simulink model "INVERTER_Arduino"  (R2022b)
settings: Solver=FixedStepAuto  StartTime=0.0  StopTime=100e-3  FixedStep=samplerate  RelTol=1e-3  EnableMultiTasking=on
InitFcn:
  | addpath('Library_Subsystems')
  | 
  | samplerate = 10e-3;
  | samplerate_serial = 100e-3;
  | samplerate_udp = 100e-3;
  | 
  | fsw = 10000;
  | 
  | 
  | PWMclock = 100e6;
  | period = PWMclock/fsw/2;
libraries: arduinolib x3, simulink x2
settings Model: SimulationMode=external  ExtModeTrigDuration=2  Creator=ReiterTo  LastModifiedBy=ReiterTo
settings SolverCC: AlgebraicLoopSolver=TrustRegion  PositivePriorityOrder=on  AutoInsertRateTranBlk=on
settings DataIOCC: LimitDataPoints=on  MaxDataPoints=10000  InspectSignalLogs=on
settings OptimizationCC: DefaultParameterBehavior=Inlined  GainParamInheritBuiltInType=on  UseFloatMulNetSlope=on  InlineInvariantSignals=on  EnhancedBackFolding=on  StrengthReduction=on  PassReuseOutputArgsAs=Individual arguments  ZeroExternalMemoryAtStartup=off  ZeroInternalMemoryAtStartup=off  NoFixptDivByZeroProtection=on  EfficientFloat2IntCast=on  LifeSpan=1  MaxStackSize=64  BufferReusableBoundary=off  OptimizeBlockOrder=speed  OptimizationPriority=Speed  MultiThreadedLoops=on  EfficientTunableParamExpr=on
settings DebuggingCC: ParameterOverflowMsg=none  ParameterUnderflowMsg=error  ParameterPrecisionLossMsg=none  ParameterTunabilityLossMsg=error
settings HardwareCC: ProdBitPerPointer=32  ProdBitPerSizeT=32  ProdBitPerPtrDiffT=32  ProdLargestAtomicInteger=Long  ProdLargestAtomicFloat=Double  ProdWordSize=32  ProdHWDeviceType=ARM Compatible->ARM Cortex  UseEmbeddedCoderFeatures=off
settings SFSimCC: MATLABDynamicMemAlloc=off
settings RTWCC: Description=Embedded Coder  SystemTargetFile=ert.tlc  HardwareBoard=Arduino Nano 33 IoT  TLCOptions=-aInlineSetEventsForThisBaseRateFcn=TLC_FALSE -aSuppressMultiTaskScheduler=TLC_FALSE -aRateBasedStepFcn=1  TemplateMakefile=ert_default_tmf  Toolchain=Arduino ARM  BuildConfiguration=Faster Runs  CodeProfilingSaveOptions=MetricsOnly
settings CodeAppCC: ForceParamTrailComments=on  IgnoreCustomStorageClasses=off  OperatorAnnotations=on  SimulinkDataObjDesc=on  SFDataObjDesc=on  InsertBlockDesc=on
settings ERTTargetCC: TargetLangStandard=C99 (ISO)  SupportNonFinite=off  SupportNonInlinedSFcns=on  SupportVariableSizeSignals=on  ExtModeTransport=3  ExtModeStaticAlloc=on  ExtModeStaticAllocSize=8192  ExtModeMexFile=ext_xcp  ExtModeIntrfLevel=Level2 - Open

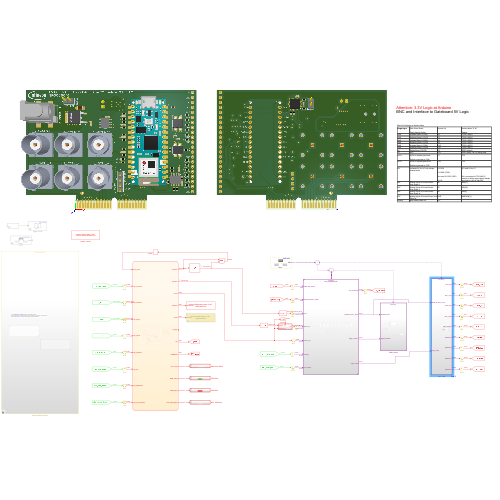
[thumbnail: Simulink's stored preview of the top-level diagram]
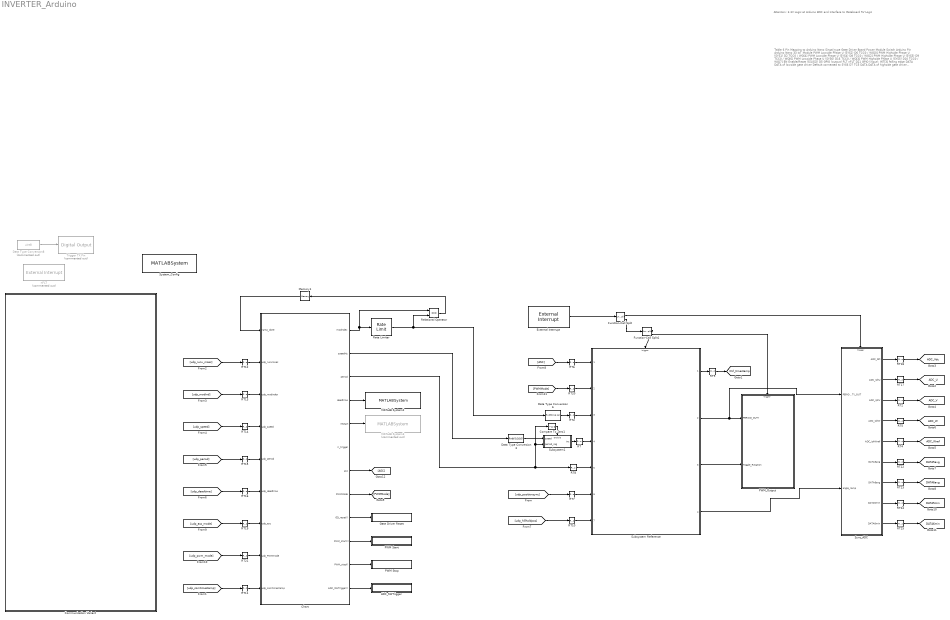
== system INVERTER_Arduino ==
  note: Attention: 3.3V Logic at Arduino
      | BNC and Interface to Gateboard 5V Logic
  note: Table 6 Pin Mapping to Arduino Nano
      | Singal type
      | Gate Driver Board
      | Power Module Switch
      | Arduino Pin
      |
      | Arduino Nano 33 IoT
      | Module
      |
      | PWM
      | Lowside Phase U (SYS2)
      | D6
      | TCC0 / WO[0]
      |
      | PWM
      | Highside Phase U (SYS1)
      | D2
      | TCC0 / WO[4]
      |
      | PWM
      | Lowside Phase U (SYS4)
      | D8
      | TCC0 / WO[2]
      |
      | PWM
      | Highside Phase U (SYS3)
      | D9
      | TCC0 / WO[6]
      |
      | PWM
      | Lowside Phase U (SYS6)
      | D16
      | TCC0 / WO[3]
      |
      | PWM
      | Highside Phase U (SYS5)
      | D10
      | TCC0 / WO[7]
      |
      | EN
      | Enable/Reset (SI1|SI2)
      | D5
      | GPIO (output)
      |
      | FLT
      | nFLT
      | D21
      | GPIO (input); INT[3] falling edge
      |
      | DATA
      | DATA of lowside gate driver
      | Default connected to SYS6
      | D7
      | TC5
      |
      | DATA
      | DATA of highside gate driver
      | Default connected to SYS5
      | D15
      | TC4
      |
      | SPI
      | Isolated ADC for DC-Link voltage measurement
      | D13 SCK
      | D12 SDO (CIPO)
      | Not used D11 SDI (COPI)
      | D4 CS
      | SPI with D4 for CS
      |
      | D4 is connected to TCC1/WO[1] module. A falling edge triggers sample and hold for the HV side ADC
      |
      | ADC
      | Analog Signal of Current Sensor Aout Phase U
      | A6
      | AIN[17]
      |
      | ADC
      | Analog Signal of Current Sensor Aout Phase V
      | A3
      | AIN[18]
      |
      | ADC
      | Analog Signal of Current Sensor Aout Phase W
      | A0
      | AIN[0]
      |
      | ADC
      | Analog Signal of Current Sensor Vref Phase W
      | AREF
      | AREF/AIN[1]
      |
      | Memory
      | Non volatile FRAM I2C
      | I2C
  ADC_SWTrigger : Subsystem  TreatAsAtomicUnit=on
  Chart : Stateflow chart  TreatAsAtomicUnit=on
  Communication Variant : Subsystem  Variant=on  VariantControlMode=label  LabelModeActiveChoice=Communicate_CodeGen
  Compare To Zero1 : simulink/Logic and Bit Operations/Compare To Zero  relop=~=  OutDataTypeStr=boolean
  Data Type Conversion3 : DataTypeConversion  OutDataTypeStr=fixdt(0,16,6)  SaturateOnIntegerOverflow=off  RndMeth=Floor
  Data Type Conversion6 : DataTypeConversion  OutDataTypeStr=fixdt(0,16,14)  SaturateOnIntegerOverflow=off  RndMeth=Floor
  Data Type Conversion8 : DataTypeConversion  Commented=on  OutDataTypeStr=uint8  SaturateOnIntegerOverflow=off  RndMeth=Floor
  External Interrupt : arduinolib/External Interrupt  Pin=3  PullUp=off  Mode=FALLING  InterruptSimulationInput=off
  Function-Call Split : FunctionCallSplit  NumOutputPorts=2  OutputPortLayout=default
  Function-Call Split1 : FunctionCallSplit  NumOutputPorts=2
  Gate Driver Reset : Subsystem  TreatAsAtomicUnit=on
  MATLAB System2 : MATLABSystem  System=invPWM_DeadTime
      mask Type: invPWM_DeadTime
      mask Display:
      | disp('Inverter PWM Arduino Nano 33 IoT \n PWM DeadTime');
      | port_label('input',1,'DeadTime');
  MATLAB System3 : MATLABSystem  Commented=on  System=invWatchDog
      mask Type: invWatchDog
      mask Display:
      | disp('Inverter Arduino Nano 33 IoT \n System Restart');
      | port_label('input',1,'Restart');
  Memory1 : Memory  InheritSampleTime=on  LinearizeMemory=on  StateName=ctrl_timestamp_z1
  PWM Start : Subsystem  TreatAsAtomicUnit=on
  PWM Stop : Subsystem  TreatAsAtomicUnit=on
  PWM_Output : Subsystem
  RT{,3,6..8,10,20} (7 alike) : RateTransition  Deterministic=off
  RT{2,4..5,11..19,21} (13 alike) : RateTransition  Deterministic=off  OutPortSampleTime=samplerate
  RT{9,22..25} (5 alike) : RateTransition  Integrity=off  Deterministic=off  OutPortSampleTime=samplerate
  Rate Limiter : RateLimiter  RisingSlewLimit=2  FallingSlewLimit=-2  SampleTimeMode=inherited
  Relational Operator : RelationalOperator  Operator===  OutDataTypeStr=boolean  RndMeth=Simplest  InputSameDT=off
  Subsystem Reference : Subsystem  InitFcn=load('PWMLookUp.mat');  RTWFileName=PWMGeneration  ReferencedSubsystem=INV_PWMsyncTask
      settings: RTWFileNameOpts=User specified
  Subsystem1 : Subsystem
  Sync_ADC : Subsystem
  System_Config : MATLABSystem  Priority=1  System=invClockGen
      mask Type: invClockGen
      mask Display: disp('Inverter Arduino Nano 33 IoT \n Generic Glock Generator Init');
  Trigger TX Pin : arduinolib/Digital Output  Commented=on  pinNumber=1  Direction=output  blockPlatform=arduino
  nFLT : arduinolib/External Interrupt  Commented=on  Pin=21  PullUp=on  Mode=FALLING  InterruptSimulationInput=off
  tag scope: ADC_U=global, ADC_V=global, ADC_Vdc=global, ADC_W=global, ADC_Wref=global, Ctrl_timestamp=global, DATA5avg=global, DATA5min=global, DATA6avg=global, DATA6min=global
  wires:
  Chart/2(speedHz) -> Data Type Conversion3/1
  Data Type Conversion6/1 -> RT3/1
  Rate Limiter/1 -> Data Type Conversion6/1, Relational Operator/2
  Sync_ADC/2(ADC_IphU) -> RT17/1
  RT8/1 -> Subsystem Reference/5
  RT9/1 -> [Ctrl_timestamp]
  Subsystem Reference/1 -> RT9/1
  RT3/1 -> Subsystem Reference/3
  RT11/1 -> Chart/9(udp_comtimestamp)
  [udp_comtimestamp] -> RT11/1
  RT12/1 -> Chart/2(udp_runxmsec)
  [udp_runx_msec] -> RT12/1
  RT13/1 -> Chart/3(udp_modindex)
  [udp_modind] -> RT13/1
  RT14/1 -> Chart/4(udp_speed)
  [udp_speed] -> RT14/1
  RT15/1 -> Chart/5(udp_period)
  [udp_period] -> RT15/1
  RT16/1 -> Chart/6(udp_deadtime)
  [udp_deadtime] -> RT16/1
  RT17/1 -> [ADC_U]
  RT18/1 -> [ADC_Vdc]
  Sync_ADC/1(ADC_SPI) -> RT18/1
  Chart/4(deadtime) -> MATLAB System2/1
  Chart/5(restart) -> MATLAB System3/1
  RT2/1 -> [ADC_V]
  Sync_ADC/3(ADC_IphV) -> RT2/1
  Sync_ADC/5(ADC_IphWref) -> RT4/1
  RT4/1 -> [ADC_Wref]
  Function-Call Split/1 -> Sync_ADC/Trigger
  RT5/1 -> [ADC_W]
  Sync_ADC/4(ADC_IphW) -> RT5/1
  Data Type Conversion8/1 -> Trigger TX Pin/1
  Chart/9(GD_reset()) -> Gate Driver Reset/Trigger
  Chart/10(PWM_start()) -> PWM Start/Trigger
  Chart/11(PWM_stop()) -> PWM Stop/Trigger
  Relational Operator/1 -> Memory1/1
  Chart/1(modindex) -> Rate Limiter/1, Relational Operator/1
  Memory1/1 -> Chart/1(ramp_done)
  RT6/1 -> Subsystem Reference/1
  [udp_positionsync] -> RT7/1
  RT7/1 -> Subsystem Reference/6
  [udp_hillholdpos] -> RT10/1
  RT10/1 -> Subsystem Reference/7
  Chart/7(asc) -> [ASC]
  [udp_asc_mode] -> RT19/1
  [ASC] -> RT6/1
  RT19/1 -> Chart/7(udp_asc)
  RT20/1 -> Subsystem Reference/2
  RT21/1 -> Chart/8(udp_PWMmode)
  [udp_pwm_mode] -> RT21/1
  Chart/8(PWMMode) -> [PWMMode]
  [PWMMode] -> RT20/1
  Chart/3(period) -> Compare To Zero1/1, Subsystem1/2(period_reg), RT8/1
  Compare To Zero1/1 -> Subsystem1/Enable
  Data Type Conversion3/1 -> Subsystem1/1(speed)
  Subsystem1/1(inc) -> RT/1
  RT/1 -> Subsystem Reference/4
  Sync_ADC/6(DATA5avg) -> RT22/1
  Sync_ADC/7(DATA6avg) -> RT23/1
  Sync_ADC/8(DATA5min) -> RT24/1
  Sync_ADC/9(DATA6min) -> RT25/1
  RT22/1 -> [DATA5avg]
  RT23/1 -> [DATA6avg]
  RT24/1 -> [DATA5min]
  RT25/1 -> [DATA6min]
  Chart/12(ADC_SWTrigger()) -> ADC_SWTrigger/Trigger
  Function-Call Split/2 -> Function-Call Split1/1
  Function-Call Split1/1 -> Subsystem Reference/Trigger
  Function-Call Split1/2 -> PWM_Output/Trigger
  Subsystem Reference/4 -> Sync_ADC/2(angle_ramp)
  Subsystem Reference/2 -> Sync_ADC/1(PERIOD_DUTY_OUT), PWM_Output/1(PERIOD_DUTY)
  Subsystem Reference/3 -> PWM_Output/2(Toggle_Rotation)
  External Interrupt/1 -> Function-Call Split/1

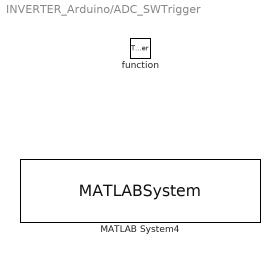
== system INVERTER_Arduino/ADC_SWTrigger ==
  function : TriggerPort  TriggerType=function-call  VariantControl=(inherit)
  MATLAB System4 : MATLABSystem  System=invADC_usertrigger
      mask Type: invADC_usertrigger
      mask Display: disp('Inverter ADC Trigger from User Event');

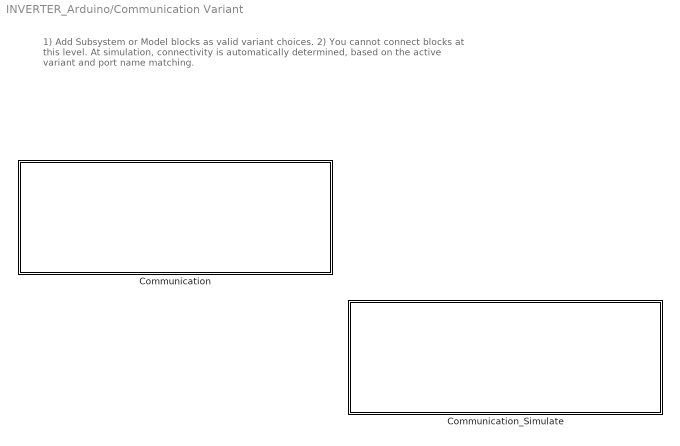
== system INVERTER_Arduino/Communication Variant ==
  note: 1) Add Subsystem or Model blocks as valid variant choices.
      | 2) You cannot connect blocks at this level. At simulation, connectivity is automatically
      | determined, based on the active variant and port name matching.
  Communication : Subsystem  VariantControl=Communicate_CodeGen  ReferencedSubsystem=Communication
  Communication_Simulate : Subsystem  VariantControl=Communicate_SimulationOnly  ReferencedSubsystem=Communication_Simulate

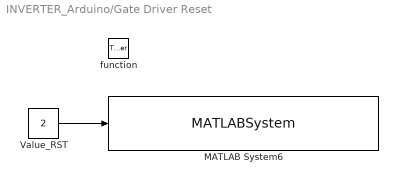
== system INVERTER_Arduino/Gate Driver Reset ==
  function : TriggerPort  TriggerType=function-call  VariantControl=(inherit)
  MATLAB System6 : MATLABSystem  System=invGD_reset
      mask Type: invGD_reset
      mask Display:
      | disp('Inverter PWM Arduino Nano 33 IoT \n GATE DRIVER RESET');
      | port_label('input',1,'rst_status');
  Value_RST : Constant  Value=2  OutDataTypeStr=uint8  SampleTime=-1
  wires:
  Value_RST/1 -> MATLAB System6/1

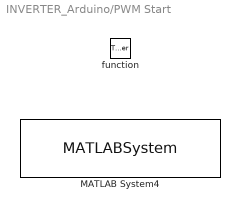
== system INVERTER_Arduino/PWM Start ==
  function : TriggerPort  TriggerType=function-call  VariantControl=(inherit)
  MATLAB System4 : MATLABSystem  System=invPWM_Start
      mask Type: invPWM_Start
      mask Display: disp('Inverter PWM Arduino Nano 33 IoT \n PWM START');

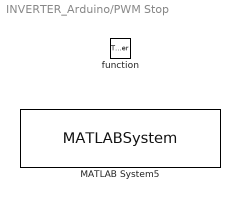
== system INVERTER_Arduino/PWM Stop ==
  function : TriggerPort  TriggerType=function-call  VariantControl=(inherit)
  MATLAB System5 : MATLABSystem  System=invPWM_Stop
      mask Type: invPWM_Stop
      mask Display: disp('Inverter PWM Arduino Nano 33 IoT \n PWM STOP');

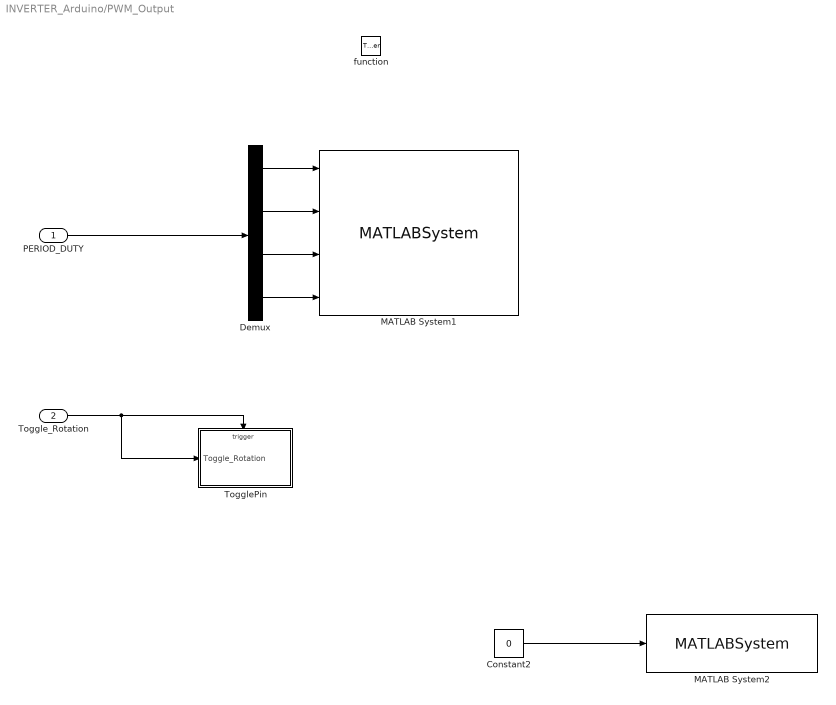
== system INVERTER_Arduino/PWM_Output ==
  PERIOD_DUTY : Inport
  Toggle_Rotation : Inport  Port=2
  function : TriggerPort  TriggerType=function-call  VariantControl=(inherit)
  Constant2 : Constant  Value=0  OutDataTypeStr=uint8  SampleTime=-1
  Demux : Demux
  MATLAB System1 : MATLABSystem  Priority=90  System=invPWM_DutyPeriod
      mask Type: invPWM_DutyPeriod
      mask Display:
      | disp('Inverter PWM Arduino Nano 33 IoT');
      | port_label('input',1,'Period');
      | port_label('input',2,'Du');
      | port_label('input',3,'Dv');
      | port_label('input',4,'Dw');
  MATLAB System2 : MATLABSystem  Priority=100  System=invIOfastRX1
      mask Type: invIOfastRX1
      mask Display:
      | disp('Arduino Nano 33 IoT \n IO 1 RX FAST');
      | port_label('input',1,'level');
  TogglePin : Subsystem  Priority=95  TreatAsAtomicUnit=on
  wires:
  PERIOD_DUTY/1 -> Demux/1
  Demux/4 -> MATLAB System1/4
  Demux/3 -> MATLAB System1/3
  Demux/2 -> MATLAB System1/2
  Demux/1 -> MATLAB System1/1
  Toggle_Rotation/1 -> TogglePin/1(Toggle_Rotation), TogglePin/Trigger
  Constant2/1 -> MATLAB System2/1

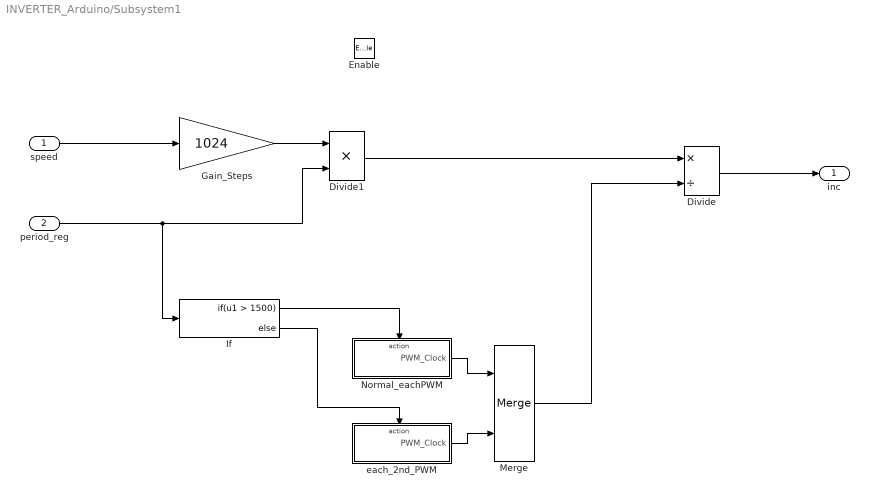
== system INVERTER_Arduino/Subsystem1 ==
  speed : Inport
  period_reg : Inport  Port=2
  Enable : EnablePort
  Divide : Product  Inputs=*/  OutDataTypeStr=fixdt(0,32,16)  RndMeth=Simplest
  Divide1 : Product  Inputs=**  OutDataTypeStr=uint32  RndMeth=Simplest
  Gain_Steps : Gain  Gain=1024  ParamDataTypeStr=int32  OutDataTypeStr=uint32  RndMeth=Simplest  LockScale=on
  If : If  IfExpression=u1 > 1500
  Merge : Merge
  Normal_eachPWM : Subsystem  TreatAsAtomicUnit=on
  each_2nd_PWM : Subsystem  TreatAsAtomicUnit=on
  inc : Outport
  wires:
  speed/1 -> Gain_Steps/1
  Merge/1 -> Divide/2
  Gain_Steps/1 -> Divide1/1
  Divide1/1 -> Divide/1
  Divide/1 -> inc/1
  period_reg/1 -> If/1, Divide1/2
  If/1 -> Normal_eachPWM/Action
  If/2 -> each_2nd_PWM/Action
  Normal_eachPWM/1(PWM_Clock) -> Merge/1
  each_2nd_PWM/1(PWM_Clock) -> Merge/2

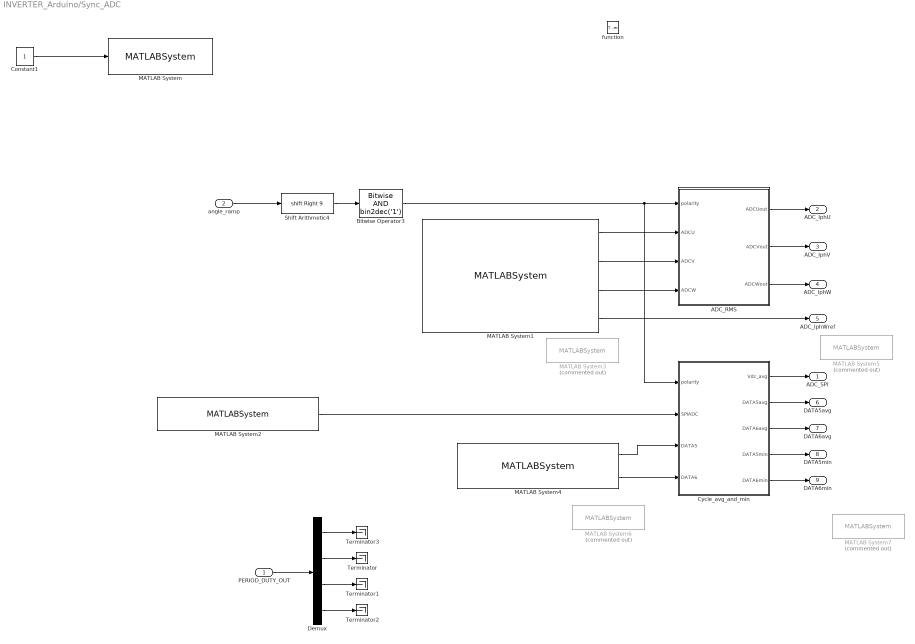
== system INVERTER_Arduino/Sync_ADC ==
  PERIOD_DUTY_OUT : Inport
  angle_ramp : Inport  Port=2
  function : TriggerPort  TriggerType=function-call  VariantControl=(inherit)
  ADC_RMS : Stateflow chart  Priority=20  TreatAsAtomicUnit=on
      settings: RTWSystemCode=Reusable function  RTWFileNameOpts=Use subsystem name
  Bitwise Operator3 : simulink/Logic and Bit Operations/Bitwise Operator  logicop=AND  UseBitMask=on  BitMask=bin2dec('1')  BitMaskRealWorld=Stored Integer
  Constant1 : Constant  Priority=1  OutDataTypeStr=uint8  SampleTime=-1
  Cycle_avg_and_min : Stateflow chart  Priority=40  TreatAsAtomicUnit=on
      settings: RTWSystemCode=Reusable function  RTWFileNameOpts=Use subsystem name
  Demux : Demux
  MATLAB System : MATLABSystem  Priority=0  System=invIOfastRX1
      mask Type: invIOfastRX1
      mask Display:
      | disp('Arduino Nano 33 IoT \n IO 1 RX FAST');
      | port_label('input',1,'level');
  MATLAB System1 : MATLABSystem  Priority=10  System=invADC
      mask Type: invADC
      mask Display:
      | disp('Inverter ADC Arduino Nano 33 IoT');
      | port_label('output',1,'ADC_IphU');
      | port_label('output',2,'ADC_IphV');
      | port_label('output',3,'ADC_IphW');
      | port_label('output',4,'ADC_IrefW');
  MATLAB System2 : MATLABSystem  Priority=1  System=invDMASPI
      mask Type: invDMASPI
      mask Display:
      | disp('Inverter DMA SPI Arduino Nano 33 IoT');
      | port_label('output',1,'DCL_RAW');
  MATLAB System3 : MATLABSystem  Priority=15  Commented=on  System=invIOfastRX1_TOGGLE
      mask Type: invIOfastRX1_TOGGLE
      mask Display: disp('Arduino Nano 33 IoT \n IO 1 RX FAST TOGGLE');
  MATLAB System4 : MATLABSystem  Priority=30  System=invCAPTURE
      mask Type: invCAPTURE
      mask Display:
      | disp('Inverter TC Capture Arduino Nano 33 IoT');
      | port_label('output',1,'DATA5');
      | port_label('output',2,'DATA6');
  MATLAB System5 : MATLABSystem  Priority=25  Commented=on  System=invIOfastRX1_TOGGLE
      mask Type: invIOfastRX1_TOGGLE
      mask Display: disp('Arduino Nano 33 IoT \n IO 1 RX FAST TOGGLE');
  MATLAB System6 : MATLABSystem  Priority=35  Commented=on  System=invIOfastRX1_TOGGLE
      mask Type: invIOfastRX1_TOGGLE
      mask Display: disp('Arduino Nano 33 IoT \n IO 1 RX FAST TOGGLE');
  MATLAB System7 : MATLABSystem  Priority=100  Commented=on  System=invIOfastRX1_TOGGLE
      mask Type: invIOfastRX1_TOGGLE
      mask Display: disp('Arduino Nano 33 IoT \n IO 1 RX FAST TOGGLE');
  Shift Arithmetic4 : ArithShift  BitShiftNumber=9  BitShiftDirection=Right
  Terminator{,1..3} (4 alike) : Terminator
  ADC_SPI : Outport
  ADC_IphU : Outport  Port=2
  ADC_IphV : Outport  Port=3
  ADC_IphW : Outport  Port=4
  ADC_IphWref : Outport  Port=5
  DATA5avg : Outport  Port=6
  DATA6avg : Outport  Port=7
  DATA5min : Outport  Port=8
  DATA6min : Outport  Port=9
  wires:
  Bitwise Operator3/1 -> Cycle_avg_and_min/1(polarity), ADC_RMS/1(polarity)
  MATLAB System4/1 -> Cycle_avg_and_min/3(DATA5)
  MATLAB System4/2 -> Cycle_avg_and_min/4(DATA6)
  Cycle_avg_and_min/2(DATA5avg) -> DATA5avg/1
  Cycle_avg_and_min/3(DATA6avg) -> DATA6avg/1
  Cycle_avg_and_min/4(DATA5min) -> DATA5min/1
  Cycle_avg_and_min/5(DATA6min) -> DATA6min/1
  Cycle_avg_and_min/1(Vdc_avg) -> ADC_SPI/1
  Constant1/1 -> MATLAB System/1
  MATLAB System1/2 -> ADC_RMS/3(ADCV)
  MATLAB System1/1 -> ADC_RMS/2(ADCU)
  MATLAB System1/3 -> ADC_RMS/4(ADCW)
  ADC_RMS/1(ADCUout) -> ADC_IphU/1
  ADC_RMS/2(ADCVout) -> ADC_IphV/1
  MATLAB System1/4 -> ADC_IphWref/1
  ADC_RMS/3(ADCWout) -> ADC_IphW/1
  Shift Arithmetic4/1 -> Bitwise Operator3/1
  angle_ramp/1 -> Shift Arithmetic4/1
  Demux/2 -> Terminator/1
  Demux/3 -> Terminator1/1
  Demux/1 -> Terminator3/1
  PERIOD_DUTY_OUT/1 -> Demux/1
  Demux/4 -> Terminator2/1
  MATLAB System2/1 -> Cycle_avg_and_min/2(SPIADC)

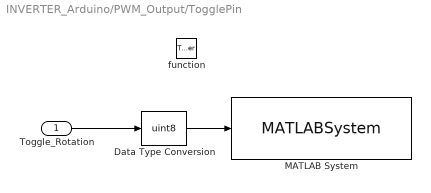
== system INVERTER_Arduino/PWM_Output/TogglePin ==
  Toggle_Rotation : Inport
  function : TriggerPort  TriggerType=either  VariantControl=(inherit)
  Data Type Conversion : DataTypeConversion  OutDataTypeStr=uint8  RndMeth=Simplest  SaturateOnIntegerOverflow=off
  MATLAB System : MATLABSystem  System=invIOfastTX0
      mask Type: invIOfastTX0
      mask Display:
      | disp('Arduino Nano 33 IoT \n IO 0 TX FAST');
      | port_label('input',1,'level');
  wires:
  Data Type Conversion/1 -> MATLAB System/1
  Toggle_Rotation/1 -> Data Type Conversion/1

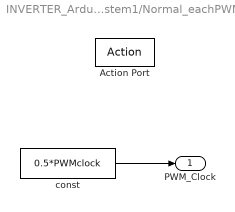
== system INVERTER_Arduino/Subsystem1/Normal_eachPWM ==
  Action Port : ActionPort  ActionPortLabel=if(u1 > 1500)
  const : Constant  Value=0.5*PWMclock  OutDataTypeStr=uint32
  PWM_Clock : Outport
  wires:
  const/1 -> PWM_Clock/1

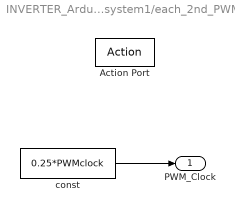
== system INVERTER_Arduino/Subsystem1/each_2nd_PWM ==
  Action Port : ActionPort  ActionPortLabel=else
  const : Constant  Value=0.25*PWMclock  OutDataTypeStr=uint32
  PWM_Clock : Outport
  wires:
  const/1 -> PWM_Clock/1

== stateflow chart INVERTER_Arduino/Sync_ADC/Cycle_avg_and_min ==
  state DETECT_POLARITY [parallel]
    settings: executionOrder=1
    state CYCLE_RESET
      en: i = uint16(0);
      en:DATA5avgbuf = uint32(0);
      en:DATA6avgbuf = uint32(0);
      en:Vdc_avgbuf = uint32(0);
      en:DATA5minbuf=uint16(0xFFFF);
      en:DATA6minbuf=uint16(0xFFFF);
    (default) -> CYCLE_RESET
    (junction 96) -> CYCLE_RESET : [i>0]
        | {
        | %DATA5avg=DATA5avgbuf/i;
        | %DATA6avg=DATA6avgbuf/i;
        | %Vdc_avg=Vdc_avgbuf/i;
        | i_resbuf=i;
        | DATA5resbuf = DATA5avgbuf;
        | DATA6resbuf = DATA6avgbuf;
        | Vdc_resbuf = Vdc_avgbuf;
        | send(CALC_OUTPUT,AVG_Output);
        |
        | DATA5min=DATA5minbuf;
        | DATA6min=DATA6minbuf;
        | }
    CYCLE_RESET -> (junction 96) : [hasChangedTo(polarity,0)|(i>10000)]
  state AVG [parallel]
    settings: executionOrder=2
    state SUMUP
      i = i+1;
      DATA5avgbuf = DATA5avgbuf + uint32(DATA5);
      DATA6avgbuf = DATA6avgbuf + uint32(DATA6);
      Vdc_avgbuf = Vdc_avgbuf + uint32(SPIADC);
    (default) -> SUMUP
  state AVG_Output [parallel]
    settings: executionOrder=5
    state WAIT_RESULTREADY
    state RESULT_n
    state RESULT1
      en:DATA5avg=DATA5resbuf/i_resbuf;
    state RESULT2
      en:DATA6avg=DATA6resbuf/i_resbuf;
    state RESULT3
      en:Vdc_avg=Vdc_resbuf/i_resbuf;
    (default) -> WAIT_RESULTREADY
    WAIT_RESULTREADY -> RESULT_n : CALC_OUTPUT
    RESULT3 -> WAIT_RESULTREADY
    RESULT_n -> RESULT1
    RESULT1 -> RESULT2
    RESULT2 -> RESULT3
  state MIN5 [parallel]
    settings: executionOrder=3
    state TESTMIN5
    (default) -> TESTMIN5
    TESTMIN5 -> TESTMIN5 : [DATA5minbuf>DATA5]{DATA5minbuf = DATA5;}
  state MIN6 [parallel]
    settings: executionOrder=4
    state TESTMIN6
    (default) -> TESTMIN6
    TESTMIN6 -> TESTMIN6 : [DATA6minbuf>DATA6]{DATA6minbuf = DATA6;}
  data: Vdc_avg output uint16 size=1 =uint16(0); polarity input uint16 size=1 =uint32(0); SPIADC input uint16 size=1; DATA5 input uint16 size=1; DATA5avg output uint16 size=1 =uint16(0); DATA6 input uint16; DATA6avg output uint16 size=1 =uint16(0); DATA5min output uint16 size=1 =uint16(0); DATA6min output uint16 size=1 =uint16(0); DATA5avgbuf local uint32 size=1 =uint32(0); DATA6avgbuf local uint32 size=1 =uint32(0); DATA5minbuf local uint16 size=1 =uint16(0xFFFF); DATA6minbuf local uint16 size=1 =uint16(0xFFFF); i local uint16 size=1 =uint16(0); Vdc_avgbuf local uint32 size=1 =uint32(0); DATA5resbuf local uint32 size=1 =uint32(0); DATA6resbuf local uint32 size=1 =uint32(0); Vdc_resbuf local uint32 size=1 =uint32(0); i_resbuf local uint16 size=1 =uint16(0)
  events: CALC_OUTPUT local FUNCTION_CALL_EVENT

== stateflow chart INVERTER_Arduino/Chart ==
  state CONTROL_STATEFLOW [parallel]
    settings: executionOrder=1
    state GD_RESET
      en: send(GD_reset);
      en: speedHz = 500; %default before run
      en: period = 5000; %default before run
      en: deadtime = 50; %default before run
      en: asc = 0;
      en: PWMMode = 0; %SVPWM
    state Standby
      ir_trigger = 0;
      en: send(PWM_stop);
      en: modindex = 0;
      ex: send(GD_reset);
      en: asc = 0;
      en: PWMMode = 0; %SVPWM
      du: send(ADC_SWTrigger);
    state Prep_directCtrl
      modindex = udp_modindex;
      speedHz = udp_speed;
      period = udp_period;
      deadtime = udp_deadtime;
      en: PWMMode = uint8(udp_PWMmode);
      ex: send(PWM_start);
    state Start_Run1
      en: xmsec=udp_runxmsec;
      en: modindex = udp_modindex;
      en: speedHz = udp_speed;
      en: period = udp_period;
      en: deadtime = udp_deadtime;
      en: PWMMode = uint8(udp_PWMmode);
      ex: send(PWM_start);
    state Run_directCtrl
      modindex = udp_modindex;
      speedHz = udp_speed;
      period = udp_period;
      deadtime = udp_deadtime;
      PWMMode = uint8(udp_PWMmode);
    state Rampup
    state PWM_SteadyState
    state ASC
      en: asc = uint8(udp_asc);
    state Rampdown
      en: modindex = 0;
    state Stop
      en: send(PWM_stop);
      en: modindex = 0;
    (default) -> GD_RESET
    GD_RESET -> Standby
    Standby -> (junction 53) : [udp_runxmsec ~= 0]
    Stop -> Standby : [udp_runxmsec == 0]
        | %restart only possible after user stop
    PWM_SteadyState -> Standby [order 2] : [in(EMERGENCY_STATEFLOW.EMERGENCY_STOP)]
    (junction 53) -> Prep_directCtrl [order 1] : [udp_runxmsec == 0xFFFFFFFF]
        | %use direct control when user select max uint32
    (junction 53) -> Start_Run1 [order 2]
    Prep_directCtrl -> Run_directCtrl
    Run_directCtrl -> Run_directCtrl [order 3]
    Start_Run1 -> Rampup
    Run_directCtrl -> ASC [order 2] : [udp_asc ~= 0]
    Rampup -> PWM_SteadyState : [ramp_done==1]
    Run_directCtrl -> Rampdown [order 1] : [udp_runxmsec < 0xFFFFFFFF]
        | %user has to stop
    PWM_SteadyState -> (junction 102) [order 1] : [after(xmsec*10,tick)] %avoid msec and use the 10ms sample rate
        | %stop automatic after x millisec
    (junction 102) -> ASC [order 1] : [udp_asc ~= 0]
    (junction 102) -> Rampdown [order 2]
    ASC -> Rampdown : [after(300,tick)] %avoid sec, msec and use tick to have no doubles
        | %stay 3 sec in ASC condition
    Rampdown -> Stop : [ramp_done==1]
  state EMERGENCY_STATEFLOW [parallel]
    settings: executionOrder=2
    state NORMAL
    state EMERGENCY_DETECTED
      modindex = 0;
    state EMERGENCY_STOP
      send(PWM_stop);
    state Restartrestart = 1; [commented out]
      % Attention System Restart
    (default) -> NORMAL
    EMERGENCY_STOP -> NORMAL : [(udp_comtimestamp == 0x00000001)&(udp_runxmsec == 0)]
    NORMAL -> EMERGENCY_DETECTED : [(udp_comtimestamp == 0xFFFFFFFF)&(udp_runxmsec == 0)]
    EMERGENCY_DETECTED -> EMERGENCY_STOP : [after(20,tick)]%200msec
  data: ramp_done input; modindex output fixdt(0,16,14) size=1; speedHz output fixdt(0,16,6) size=1; period output uint16 size=1 =uint16(5000); deadtime output uint8 size=1; udp_runxmsec input uint32 size=1; udp_modindex input fixdt(0,16,14) size=1; udp_speed input fixdt(0,16,6) size=1; udp_period input uint16 size=1; udp_deadtime input uint8 size=1; xmsec local uint32 size=1; restart output uint8 size=1 =uint8(0); ir_trigger output uint8 size=1 =uint8(0); asc output uint8 size=1 =uint8(0); udp_asc input uint16; udp_PWMmode input size=1; PWMMode output uint8 =uint8(0); udp_comtimestamp input uint32 size=1
  events: GD_reset output FUNCTION_CALL_EVENT; PWM_start output FUNCTION_CALL_EVENT; PWM_stop output FUNCTION_CALL_EVENT; ADC_SWTrigger output FUNCTION_CALL_EVENT

== stateflow chart INVERTER_Arduino/Sync_ADC/ADC_RMS ==
  state ADC_GetReady
  state ADC_WaitSteady
  state GETOFFSET
    i = i+1;
    ADCUbuf = ADCUbuf + int16(ADCU);
    ADCVbuf = ADCVbuf + int16(ADCV);
    ADCWbuf = ADCWbuf + int16(ADCW);
  state OFFSET
    OffsetU = ADCUbuf>>2;
    OffsetV = ADCVbuf>>2;
    OffsetW = ADCWbuf>>2;
  state SUM_UP
    en: RMSsumU = RMSsumU+((ADCU-OffsetU)*(ADCU-OffsetU));
    en: RMSsumV = RMSsumV+((ADCV-OffsetV)*(ADCV-OffsetV));
    en: RMSsumW = RMSsumW+((ADCW-OffsetW)*(ADCW-OffsetW));
  state DIV_i1
    en: RMSsumU = RMSsumU / i;
  state DIV_i2
    en: RMSsumV = RMSsumV / i;
  state Sqrt_final_value
    en: ADCUout = int16(SU);
    en: ADCVout = int16(SV);
    en: ADCWout = int16(SW);
  state DIV_i3
    en: RMSsumW = RMSsumW / i;
  state Sqrt_iterative_step11
    %iterative sqrt with NewtonRaphson Algo
    en: tmpU = (RMSsumU/SU);
  state Sqrt_iterative_step12
    %iterative sqrt with NewtonRaphson Algo
    en: tmpV = (RMSsumV/SV);
  state Sqrt_iterative_step13
    %iterative sqrt with NewtonRaphson Algo
    en: tmpW = (RMSsumW/SW);
  state Sqrt_iterative_step2
    en: SU = (SU + tmpU) >>1;
    en: SV = (SV + tmpV) >>1
    en: SW = (SW + tmpW) >>1
  (default) -> ADC_GetReady
  ADC_GetReady -> ADC_WaitSteady : [(ADCU>0)&(ADCV>0)&(ADCW>0)]
  ADC_WaitSteady -> GETOFFSET : [after(2000,tick)]%avoid 200ms as stateflow will use double value for sec
      | {i=0;}
  GETOFFSET -> OFFSET : [i==4]
  OFFSET -> (junction 176)
  Sqrt_final_value -> (junction 176)
  (junction 176) -> SUM_UP : [hasChangedTo(polarity,1)]{i=1; RMSsumU = 0; RMSsumV = 0;RMSsumW = 0;}
  SUM_UP -> SUM_UP [order 2] : {i++;}
  SUM_UP -> DIV_i1 [order 1] : [hasChangedTo(polarity,1)|(i>1000)]
      | %assumption is ratiometric output (max val 0.5*4096). Overflow will not occur before 1024
  DIV_i1 -> DIV_i2
  DIV_i2 -> DIV_i3
  Sqrt_iterative_step2 -> Sqrt_iterative_step11 [order 2] : {i++;}
  DIV_i3 -> Sqrt_iterative_step11 : {i=1;SU=1000;SV=1000;SW=1000;}
  Sqrt_iterative_step2 -> Sqrt_final_value [order 1] : [i>8]
      | %typ 7 iterations are enough
  Sqrt_iterative_step11 -> Sqrt_iterative_step12
  Sqrt_iterative_step12 -> Sqrt_iterative_step13
  Sqrt_iterative_step13 -> Sqrt_iterative_step2
  data: polarity input uint16 size=1 =uint32(0); ADCU input uint16 size=1; ADCV input uint16 size=1; ADCW input uint16 size=1 =uint16(0); ADCUout output int16 size=1 =int16(0); ADCVout output int16 size=1 =int16(0); ADCWout output int16 size=1 =int16(0); ADCUbuf local int16 size=1 =int16(0); ADCVbuf local int16 size=1 =int16(0); ADCWbuf local int16 size=1 =int16(0); OffsetV local int16 size=1 =int16(0); OffsetW local int16 size=1 =int16(0); i local uint16 size=1 =uint16(0); OffsetU local int16 size=1 =int16(0); RMSsumU local uint32 size=1 =uint32(0); RMSsumW local uint32 size=1 =uint32(0); RMSsumV local uint32 size=1 =uint32(0); tmpU local uint32 size=1 =uint32(0); SU local uint32 size=1 =uint32(0); SW local uint32 size=1 =uint32(0); SV local uint32 size=1 =uint32(0); tmpV local uint32 size=1 =uint32(0); tmpW local uint32 size=1 =uint32(0)
